simulink model "piddeffort"  (R2020a)
settings: Solver=VariableStepAuto  StartTime=0.0  StopTime=10  RelTol=1e-3
libraries: cstblocks x2
settings Model: Creator=jose  LastModifiedBy=jose

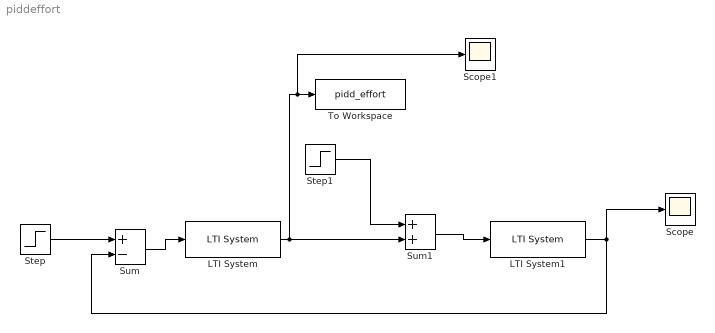
== system piddeffort ==
  LTI System : cstblocks/LTI System  sys=Cd_PIDD  IC=[]
  LTI System1 : cstblocks/LTI System  sys=Gd_d  IC=[]
  Scope : Scope
  Scope1 : Scope
  Step : Step  Time=0  After=0  SampleTime=0
  Step1 : Step  Before=1  SampleTime=0
  Sum : Sum  Inputs=+-  InputSameDT=on  SaturateOnIntegerOverflow=on  OutDataTypeStr=Inherit: Same as first input
  Sum1 : Sum  InputSameDT=on  SaturateOnIntegerOverflow=on  OutDataTypeStr=Inherit: Same as first input
  To Workspace : ToWorkspace  VariableName=pidd_effort  SaveFormat=Timeseries  SampleTime=-1
  wires:
  Step/1 -> Sum/1
  Sum/1 -> LTI System/1
  LTI System1/1 -> Scope/1, Sum/2
  Step1/1 -> Sum1/1
  Sum1/1 -> LTI System1/1
  LTI System/1 -> Sum1/2, Scope1/1, To Workspace/1
